simulink model "Model"  (R2024a)
settings: Solver=FixedStepAuto  StartTime=0.0  StopTime=0  FixedStep=0.01  RelTol=1e-3
undefined symbols (not defined in the file or in its folder): position, rotationMatrix, status, timestamp, velocity
settings Model: Creator=Scythe  LastModifiedBy=damerius
settings SolverCC: ConcurrentTasks=on
settings DataIOCC: SaveOutput=off  SignalLogging=off  DSMLogging=off  SaveTime=off  ReturnWorkspaceOutputs=off
settings OptimizationCC: DefaultParameterBehavior=Inlined  ZeroExternalMemoryAtStartup=off  ZeroInternalMemoryAtStartup=off  SimCompilerOptimization=on
settings DebuggingCC: UnconnectedInputMsg=warning  UnconnectedOutputMsg=warning  UnconnectedLineMsg=warning
settings HardwareCC: ProdBitPerLong=64  ProdHWDeviceType=Intel->x86-64 (Linux 64)
settings ModelReferenceCC: EnableRefExpFcnMdlSchedulingChecks=on
settings SFSimCC: SimParseCustomCode=off  SimGenImportedTypeDefs=on  SimTargetLang=C++
settings RTWCC: GenCodeOnly=on  PackageGeneratedCodeAndArtifacts=on  PackageName=PackNGo  RTWVerbose=off  BuildConfiguration=Faster Runs  TargetLang=C++
settings CodeAppCC: ForceParamTrailComments=on  MaxIdLength=128  StateflowObjectComments=on  MATLABSourceComments=on  UseSimReservedNames=on
settings GRTTargetCC: TargetLangStandard=C++11 (ISO)  MatFileLogging=off  CodeInterfacePackaging=C++ class

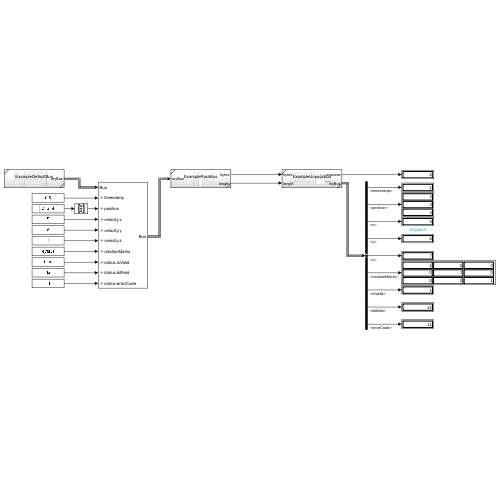
[thumbnail: Simulink's stored preview of the top-level diagram]
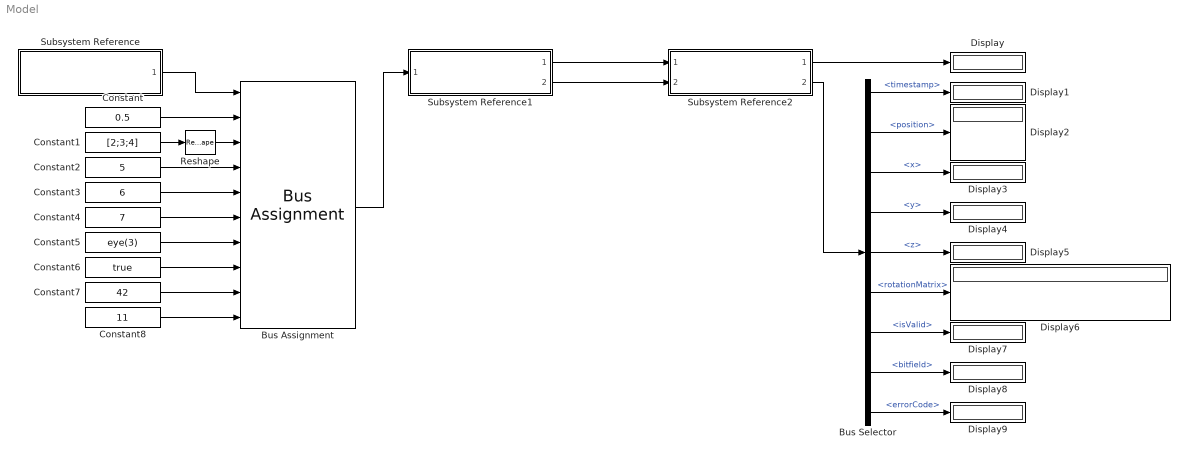
== system Model ==
  Bus Assignment : BusAssignment  AssignedSignals=timestamp,position,velocity.x,velocity.y,velocity.z,rotationMatrix,status.isValid,status.bitfield,status.errorCode
  Bus Selector : BusSelector  OutputSignals=timestamp,position,velocity.x,velocity.y,velocity.z,rotationMatrix,status.isValid,status.bitfield,status.errorCode
  Constant : Constant  Value=0.5
  Constant1 : Constant  Value=[2;3;4]
  Constant2 : Constant  Value=5  OutDataTypeStr=single
  Constant3 : Constant  Value=6  OutDataTypeStr=single
  Constant4 : Constant  Value=7  OutDataTypeStr=single
  Constant5 : Constant  Value=eye(3)
  Constant6 : Constant  Value=true  OutDataTypeStr=boolean
  Constant7 : Constant  Value=42  OutDataTypeStr=uint16
  Constant8 : Constant  Value=11  OutDataTypeStr=uint8
  Display{,1..9} (10 alike) : Display
  Reshape : Reshape  OutputDimensionality=Column vector (2-D)
  Subsystem Reference : Subsystem  ReferencedSubsystem=ExampleDefaultBus
  Subsystem Reference1 : Subsystem  ReferencedSubsystem=ExamplePackBus
  Subsystem Reference2 : Subsystem  ReferencedSubsystem=ExampleUnpackBus
  wires:
  Subsystem Reference1/1 -> Subsystem Reference2/1
  Subsystem Reference1/2 -> Subsystem Reference2/2
  Subsystem Reference/1 -> Bus Assignment/1
  Subsystem Reference2/1 -> Display/1
  Subsystem Reference2/2 -> Bus Selector/1
  Bus Selector/1 -> Display1/1  "<timestamp>"
  Bus Selector/2 -> Display2/1  "<position>"
  Constant/1 -> Bus Assignment/2
  Constant1/1 -> Reshape/1
  Constant2/1 -> Bus Assignment/4
  Constant3/1 -> Bus Assignment/5
  Constant4/1 -> Bus Assignment/6
  Constant5/1 -> Bus Assignment/7
  Constant6/1 -> Bus Assignment/8
  Constant7/1 -> Bus Assignment/9
  Constant8/1 -> Bus Assignment/10
  Bus Assignment/1 -> Subsystem Reference1/1
  Bus Selector/3 -> Display3/1  "<x>"
  Bus Selector/4 -> Display4/1  "<y>"
  Bus Selector/5 -> Display5/1  "<z>"
  Bus Selector/6 -> Display6/1  "<rotationMatrix>"
  Bus Selector/7 -> Display7/1  "<isValid>"
  Bus Selector/8 -> Display8/1  "<bitfield>"
  Bus Selector/9 -> Display9/1  "<errorCode>"
  Reshape/1 -> Bus Assignment/3
